simulink model "PM_simple_21"  (R2021b)
settings: Solver=FixedStepAuto  StartTime=0.0  StopTime=inf  RelTol=1e-3  EnableMultiTasking=on
libraries: raspberrypiCommlib x1
(part 2 of 2)

== system PM_simple_21/Run Demo ==

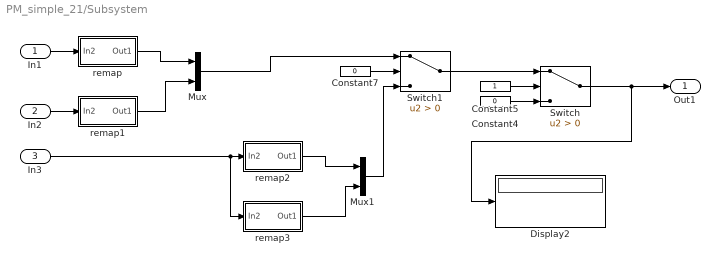
== system PM_simple_21/Subsystem ==
  In1 : Inport
  In2 : Inport  Port=2
  In3 : Inport  Port=3
  Constant4 : Constant  Value=0  OutDataTypeStr=uint8  SampleTime=1
  Constant5 : Constant  SampleTime=1
  Constant7 : Constant  Value=0  SampleTime=1
  Display2 : Display
  Mux : Mux  Inputs=2
  Mux1 : Mux  Inputs=2
  Switch : Switch  Criteria=u2 > Threshold
  Switch1 : Switch  Criteria=u2 > Threshold
  remap : Subsystem
  remap1 : Subsystem
  remap2 : Subsystem
  remap3 : Subsystem
  Out1 : Outport
  wires:
  Constant7/1 -> Switch1/2
  Mux/1 -> Switch1/1
  In3/1 -> remap3/1(In2), remap2/1(In2)
  Switch/1 -> Out1/1, Display2/1
  remap2/1(Out1) -> Mux1/1
  remap/1(Out1) -> Mux/1
  In2/1 -> remap1/1(In2)
  Mux1/1 -> Switch1/3
  Constant5/1 -> Switch/2
  remap1/1(Out1) -> Mux/2
  Constant4/1 -> Switch/3
  In1/1 -> remap/1(In2)
  remap3/1(Out1) -> Mux1/2
  Switch1/1 -> Switch/1

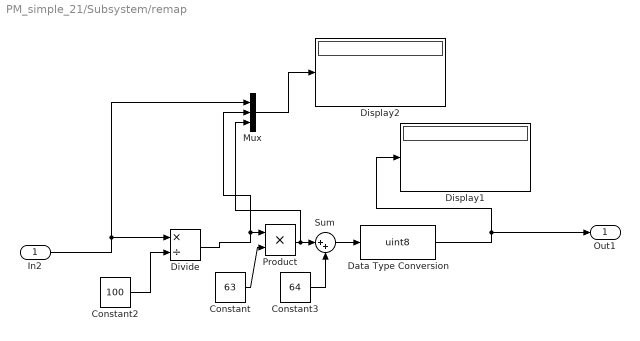
== system PM_simple_21/Subsystem/remap ==
  In2 : Inport
  Constant : Constant  Value=63
  Constant2 : Constant  Value=100  OutDataTypeStr=double
  Constant3 : Constant  Value=64  OutDataTypeStr=double
  Data Type Conversion : DataTypeConversion  OutDataTypeStr=uint8
  Display1 : Display
  Display2 : Display
  Divide : Product  Inputs=*/
  Mux : Mux  Inputs=3
  Product : Product  OutDataTypeStr=double
  Sum : Sum  Inputs=|++  OutDataTypeStr=double
  Out1 : Outport
  wires:
  Mux/1 -> Display2/1
  Constant2/1 -> Divide/2
  Data Type Conversion/1 -> Out1/1, Display1/1
  Constant/1 -> Product/2
  Product/1 -> Mux/3, Sum/1
  Sum/1 -> Data Type Conversion/1
  Constant3/1 -> Sum/2
  In2/1 -> Divide/1, Mux/1
  Divide/1 -> Mux/2, Product/1

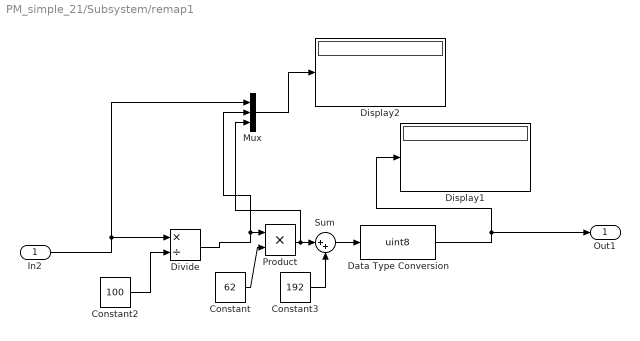
== system PM_simple_21/Subsystem/remap1 ==
  In2 : Inport
  Constant : Constant  Value=62
  Constant2 : Constant  Value=100  OutDataTypeStr=double
  Constant3 : Constant  Value=192  OutDataTypeStr=double
  Data Type Conversion : DataTypeConversion  OutDataTypeStr=uint8
  Display1 : Display
  Display2 : Display
  Divide : Product  Inputs=*/
  Mux : Mux  Inputs=3
  Product : Product  OutDataTypeStr=double
  Sum : Sum  Inputs=|++  OutDataTypeStr=double
  Out1 : Outport
  wires:
  Mux/1 -> Display2/1
  Constant2/1 -> Divide/2
  Data Type Conversion/1 -> Out1/1, Display1/1
  Constant/1 -> Product/2
  Product/1 -> Mux/3, Sum/1
  Sum/1 -> Data Type Conversion/1
  Constant3/1 -> Sum/2
  In2/1 -> Divide/1, Mux/1
  Divide/1 -> Mux/2, Product/1

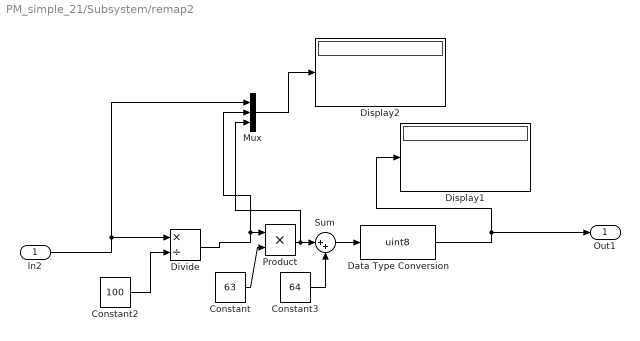
== system PM_simple_21/Subsystem/remap2 ==
  In2 : Inport
  Constant : Constant  Value=63
  Constant2 : Constant  Value=100  OutDataTypeStr=double
  Constant3 : Constant  Value=64  OutDataTypeStr=double
  Data Type Conversion : DataTypeConversion  OutDataTypeStr=uint8
  Display1 : Display
  Display2 : Display
  Divide : Product  Inputs=*/
  Mux : Mux  Inputs=3
  Product : Product  OutDataTypeStr=double
  Sum : Sum  Inputs=|++  OutDataTypeStr=double
  Out1 : Outport
  wires:
  Mux/1 -> Display2/1
  Constant2/1 -> Divide/2
  Data Type Conversion/1 -> Out1/1, Display1/1
  Constant/1 -> Product/2
  Product/1 -> Mux/3, Sum/1
  Sum/1 -> Data Type Conversion/1
  Constant3/1 -> Sum/2
  In2/1 -> Divide/1, Mux/1
  Divide/1 -> Mux/2, Product/1

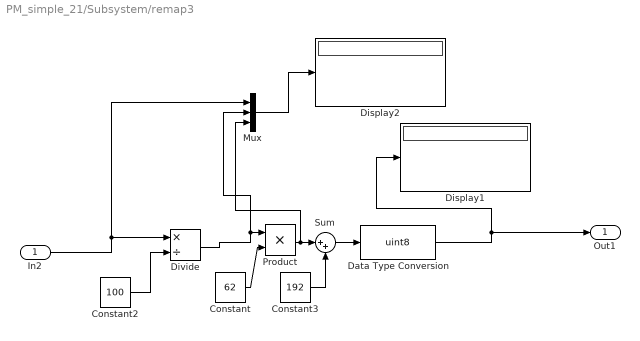
== system PM_simple_21/Subsystem/remap3 ==
  In2 : Inport
  Constant : Constant  Value=62
  Constant2 : Constant  Value=100  OutDataTypeStr=double
  Constant3 : Constant  Value=192  OutDataTypeStr=double
  Data Type Conversion : DataTypeConversion  OutDataTypeStr=uint8
  Display1 : Display
  Display2 : Display
  Divide : Product  Inputs=*/
  Mux : Mux  Inputs=3
  Product : Product  OutDataTypeStr=double
  Sum : Sum  Inputs=|++  OutDataTypeStr=double
  Out1 : Outport
  wires:
  Mux/1 -> Display2/1
  Constant2/1 -> Divide/2
  Data Type Conversion/1 -> Out1/1, Display1/1
  Constant/1 -> Product/2
  Product/1 -> Mux/3, Sum/1
  Sum/1 -> Data Type Conversion/1
  Constant3/1 -> Sum/2
  In2/1 -> Divide/1, Mux/1
  Divide/1 -> Mux/2, Product/1
